simulink model "rtdemo1"  (Simulink 7.8)
settings: Solver=FixedStepDiscrete  StartTime=0.0  StopTime=inf  FixedStep=1  RelTol=1e-3
undefined symbols (not defined in the file or in its folder): j, powergui
libraries: simulink x11, powerlib x9, CampusModeling x5, opal_lib x4, powerlib_extras x3, rtio_opalrt_op5142ex1 x3, rtlab x2
Description:
  | Model of a simple control system for use iin training.
settings Model: Creator=Paul Baracos  LastModifiedBy=wbernal  BufferReuse=off
settings DataIOCC: SaveOutput=off  SaveTime=off  SignalLoggingName=sigsOut
settings OptimizationCC: BlockReduction=off  BooleanDataType=off  InlineInvariantSignals=on  OptimizeBlockIOStorage=off  BufferReuse=off  ExpressionFolding=off  LocalBlockOutputs=off  InitFltsAndDblsToZero=on
settings DebuggingCC: SaveWithParameterizedLinksMsg=none  SignalResolutionControl=TryResolveAllWithWarning  SolverPrmCheckMsg=none  MultiTaskDSMMsg=warning  MultiTaskCondExecSysMsg=none  StrictBusMsg=None
settings HardwareCC: TargetUnknown=on
settings RTWCC: IncludeERTFirstTime=on
settings GRTTargetCC: TargetFcnLib=ansi_tfl_tmw.mat

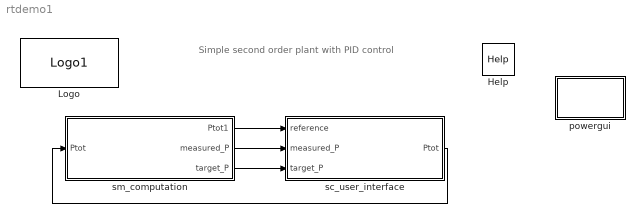
== system rtdemo1 ==
  note: Simple second order plant with PID control
  Help : opal_lib/Help  docfile=../help/help.html
  Logo : opal_lib/Logo1  vide=[]
  powergui : Subsystem  Priority=1  AncestorBlock=powerlib/powergui  InitFcn=powergui( 'InitFcn_Callback' , gcb , 0 , [ ] );  StopFcn=powergui( 'StopFcn_Callback' , gcb , 0 , [ ] );  mask(PSB option menu block){SimulationMode=Phasor, SolverType=Tustin, SampleTime=50e-6, frequency=60, SPID=off, DisableSnubberDevices=off, DisableRonSwitches=off, DisableVfSwitches=off, SwTol=0, Interpol=off, DisplayEquations=off, FunctionMessages=off, frequencyindice=60, Pbase=100e3, ErrMax=1e-4, Iterations=50, UnitsV=kV, UnitsW=MW, echomessages=off, HookPort=off, EnableUseOfTLC=off, x0status=blocks, RestoreLinks=warning, ResistiveCurrentMeasurement=off, Frange=, Ylog=off, Xlog=on, ShowGrid=off, save=off, variable=ZData, structure=, ZoomFFT=off, StartTime=0.0, cycles=1, DisplayStyle=1, fundamental=, FreqAxis=off, MaxFrequency=1000, frequencyindicesteady=1, RmsSteady=, display=off, Ts=, methode=off}
      mask prompts: SimulationMode "Simulation type:"; SolverType "Solver type:"; SampleTime "Sample time (s):"; frequency "Phasor frequency (Hz):"; SPID "Enable use of ideal switching devices"; DisableSnubberDevices "Disable snubbers in switching devices"; DisableRonSwitches "Disable On resistance in switching devices (Ron=0)"; DisableVfSwitches "Disable Forward voltage in switching devices (Vf=0)"; SwTol "Switch tolerance"; Interpol "Interpolate"; DisplayEquations "Display circuit differential equations"; FunctionMessages "Display internal function messages (debug mode feature)"; frequencyindice "Load flow frequency (Hz):"; Pbase "Base power Pbase (VA):"; ErrMax "PQ tolerance (pu):"; Iterations "Max iterations:"; UnitsV "Voltage units"; UnitsW "Power units"; echomessages "Display SimPowerSystems warnings and messages"; HookPort "Add a hook port to the powergui block"; EnableUseOfTLC "Use TLC file when in Accelerator Simulation Mode and for code generation"; x0status "Start simulation with initial electrical states from:"; RestoreLinks "Restore disabled links of SimPowerSystems blocks:"; ResistiveCurrentMeasurement "Use non ideal current measurement blocks (1e-4Ohm internal resistance)"; Frange "Frequency Range"; Ylog "Log impedance"; Xlog "log Frequency"; ShowGrid "grid"; save "Save Data To Workspace"; variable "Variable Name"; structure "Structure Name (PSBFFTSCOPE)"; ZoomFFT "ZoomFFT (PSBFFTSCOPE)"; StartTime "Start Time (PSBFFTSCOPE)"; cycles "Cycles (PSBFFTSCOPE)"; DisplayStyle "Display style (PSBFFTSCOPE)"; fundamental "Fundamental (PSBFFTSCOPE)"; FreqAxis "Frequency Axis (PSBFFTSCOPE)"; MaxFrequency "Max Frequency (PSBFFTSCOPE)"; frequencyindicesteady "Frequency indice (STEADYSTATE)"; RmsSteady "RMS display (STEADYSTATE)"; display "Display Results"; Ts "Old Ts setting (OBSOLETE)"; methode "Phasor simulation (OBSOLETE)"
      mask help: Set simulation type, simulation parameters, and preferences
      mask init:
      | message = powergui('MaskInitialization',gcb,SimulationMode,SampleTime);
      settings: CopyFcn=powergui( 'Copy_Callback' , gcb , 0 , [ ] );  ModelCloseFcn=powergui( 'CloseButton_Callback' , gcb , [ ] , [ ] );  NameChangeFcn=powergui( 'NameChangeFcn_Callback' , gcb , 0 , [ ] );  OpenFcn=powergui(gcb,'Open')
      settings: DeleteFcn=|
      | % see geck 675031 powergui( 'Copy_Callback' , gcb , 1 , [ ] );
      | 
      | powergui( 'CloseButton_Callback' , gcb , [ ] , [ ] );
      settings: PreSaveFcn=|
      | powergui( 'PreSaveFcn_Callback' , gcb , [ ] , [ ] );
      | powergui( 'CloseButton_Callback' , gcb , [ ] , [ ] );
      mask Help: helpview(psbhelp)
      mask StyleString: popup(Continuous|Discrete|Phasor),popup(Tustin|Backward Euler),edit,edit,checkbox,checkbox,checkbox,checkbox,edit,checkbox,checkbox,checkbox,edit,edit,edit,edit,popup(V|kV),popup(W|kW|MW),checkbox,checkbox,checkbox,popup(blocks|steady|zero),popup(yes|warning|no),checkbox,edit,checkbox,checkbox,checkbox,checkbox,edit,edit,checkbox,edit,edit,edit,edit,checkbox,edit,edit,edit,checkbox,edit,checkbox
      mask CallbackString: powergui('SimulationType',[],[],gcb);||||powergui('SPID',[],[],gcb);|||||||||||||||powergui('HookPort',[],[],gcb);|||||||||||||||||||||||
      mask TabNameString: Solver,Solver,Solver,Solver,Solver,Solver,Solver,Solver,Solver,Solver,Solver,Solver,Load Flow,Load Flow,Load Flow,Load Flow,Load Flow,Load Flow,Preferences,Preferences,Preferences,Preferences,Preferences,Preferences,Preferences,Preferences,Preferences,Preferences,Preferences,Preferences,Preferences,Preferences,Preferences,Preferences,Preferences,Preferences,Preferences,Preferences,Preferences,Preferences,Preferences,Solver,Solver
      mask Display: color('blue'),disp(message)
  sc_user_interface : Subsystem
  sm_computation : Subsystem
  wires:
  sc_user_interface/1(Ptot) -> sm_computation/1(Ptot)
  sm_computation/3(target_P) -> sc_user_interface/3(target_P)
  sm_computation/2(measured_P) -> sc_user_interface/2(measured_P)
  sm_computation/1(Ptot1) -> sc_user_interface/1(reference)

== system rtdemo1/powergui ==
  note: Graphical user interface for the analysis of  SimPowerSystems circuits.
      | Place the Powergui block in the top-level of your model and double-click
      | on it to open the GUI.
  EquivalentModel1 : Subsystem
      mask init:
      | SPS = get_param(gcbh,'UserData');
      | if isempty(SPS)
      | 	H=0;
      | 	Rswitch=1;
      | 	InputsNonZero=1;
      | else
      | 	H=SPS.Hswo;
      | 	Rswitch=SPS.Rswitch;
      | 	InputsNonZero=SPS.InputsNonZero;
      | end
      mask Display:
      | color('green')
      | disp('EQUIVALENT CIRCUIT\nPhasor')
  Ground : Ground
  Terminator : Terminator
  wires:
  Ground/1 -> Terminator/1

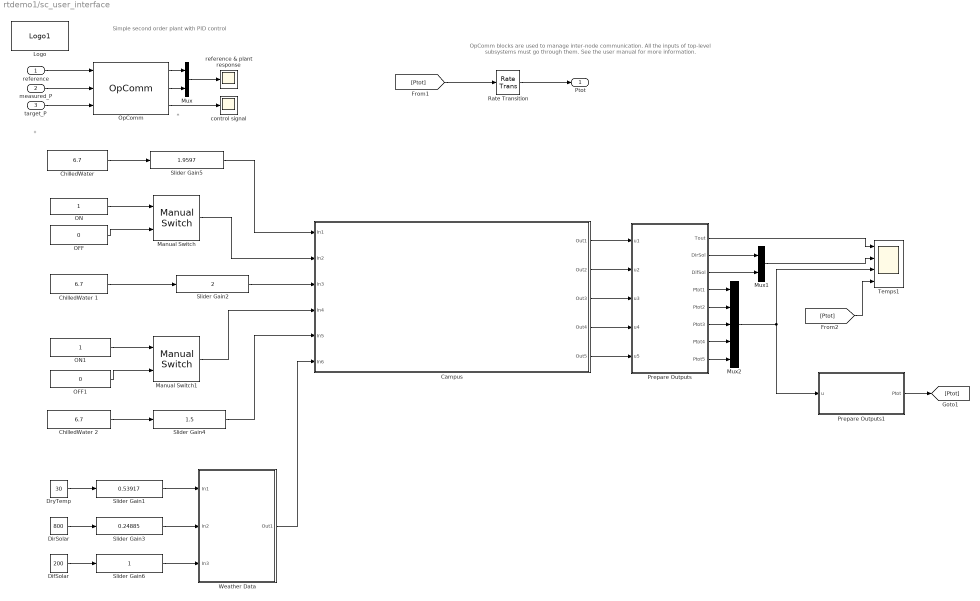
== system rtdemo1/sc_user_interface ==
  note: Simple second order plant with PID control
  note: OpComm blocks are used to manage inter-node communication. All the inputs of top-level
      | subsystems must go through them. See the user manual for more information.
  note: *
  note: *
  reference : Inport
  measured_P : Inport  Port=2
  target_P : Inport  Port=3
  Campus : Subsystem
      mask Display:
      | disp('Campus Model');
      | port_label('input', 1, 'Hospital');
      | port_label('input', 2, 'Secondary School');
      | port_label('input', 3, 'Hospital 1');
      | port_label('input', 4, 'Secondary School');
      | port_label('input', 5, 'Hospital 2');
      | 
      | port_label('output', 1, 'Pout1');
      | % port_label('input', 2, 'int');
      | % port_label('input', 3, 'bool');
      | %a = mfilename('fullpath');
      | %disp(a)
      | image(imread('Campus.jpg'))
  ChilledWater : Constant  Value=6.7
  ChilledWater 1 : Constant  Value=6.7
  ChilledWater 2 : Constant  Value=6.7
  DifSolar : Constant  Value=200
  DirSolar : Constant  Value=800
  DryTemp : Constant  Value=30
  Logo : opal_lib/Logo1  vide=[]
  Manual Switch : simulink/Signal Routing/Manual Switch  sw=0  action=0  varsize=off
  Manual Switch1 : simulink/Signal Routing/Manual Switch  sw=0  action=0  varsize=off
  Mux : Mux  Inputs=2
  Mux1 : Mux  Inputs=2
  Mux2 : Mux  Inputs=5
  OFF : Constant  Value=0
  OFF1 : Constant  Value=0
  ON : Constant
  ON1 : Constant
  OpComm : rtlab/OpComm  nbport=3  groupe_acq=1  subsys_rate=0  st=0  Synchronization=on  Interpolation=on  Threshold=1.0  Missed_Data=off  Sim_Time=off  Samples=off  dynSigOut=off  from_console=0  warning_done=off  writeOpCommFile=off  Offset=off
  Prepare Outputs : MATLAB Function  TreatAsAtomicUnit=on
  Prepare Outputs1 : MATLAB Function  TreatAsAtomicUnit=on
  Rate Transition : RateTransition
  Slider Gain1 : simulink/Math Operations/Slider Gain  low=0.5  gain=0.53917  high=1
  Slider Gain2 : simulink/Math Operations/Slider Gain  low=0.75  gain=2  high=2
  Slider Gain3 : simulink/Math Operations/Slider Gain  low=0  gain=0.24885  high=1
  Slider Gain4 : simulink/Math Operations/Slider Gain  low=0.75  gain=1.5  high=2
  Slider Gain5 : simulink/Math Operations/Slider Gain  low=0.75  gain=1.9597  high=2
  Slider Gain6 : simulink/Math Operations/Slider Gain  low=0  gain=1  high=1
  Temps1 : Scope  NumInputPorts=4
      settings: TimeRange=1883040.935672515  YMin=0~0~0~450000  YMax=21~800~425000~1.45e+006
  Weather Data : Subsystem
  control signal : Scope
      settings: YMin=609462  YMax=673616  SaveName=controlSignal
  reference & plant response : Scope
      settings: Tag=op_tm_save_it  TimeRange=10  YMin=609684  YMax=673862  SaveName=referenceAndPlant
  Ptot : Outport
  wires:
  Mux/1 -> reference & plant response/1
  reference/1 -> OpComm/1
  target_P/1 -> OpComm/3
  measured_P/1 -> OpComm/2
  OpComm/1 -> Mux/1
  OpComm/2 -> Mux/2
  OpComm/3 -> control signal/1
  Campus/1(Out1) -> Prepare Outputs/1(u1)
  Campus/2(Out2) -> Prepare Outputs/2(u2)
  Campus/3(Out3) -> Prepare Outputs/3(u3)
  Campus/4(Out4) -> Prepare Outputs/4(u4)
  Campus/5(Out5) -> Prepare Outputs/5(u5)
  Prepare Outputs/4(Ptot1) -> Mux2/1
  Prepare Outputs/5(Ptot2) -> Mux2/2
  Prepare Outputs/6(Ptot3) -> Mux2/3
  Prepare Outputs/7(Ptot4) -> Mux2/4
  Prepare Outputs/8(Ptot5) -> Mux2/5
  Manual Switch/1 -> Campus/2(In2)
  ChilledWater 1/1 -> Slider Gain2/1
  Slider Gain2/1 -> Campus/3(In3)
  ChilledWater 2/1 -> Slider Gain4/1
  Slider Gain4/1 -> Campus/5(In5)
  ChilledWater/1 -> Slider Gain5/1
  Slider Gain5/1 -> Campus/1(In1)
  ON/1 -> Manual Switch/1
  OFF/1 -> Manual Switch/2
  ON1/1 -> Manual Switch1/1
  OFF1/1 -> Manual Switch1/2
  Manual Switch1/1 -> Campus/4(In4)
  Prepare Outputs1/1(Ptot) -> [Ptot]
  Weather Data/1(Out1) -> Campus/6(In6)
  Prepare Outputs/2(DirSol) -> Mux1/1
  Prepare Outputs/3(DifSol) -> Mux1/2
  Prepare Outputs/1(Tout) -> Temps1/1
  Mux1/1 -> Temps1/2
  Mux2/1 -> Prepare Outputs1/1(u), Temps1/3
  DryTemp/1 -> Slider Gain1/1
  DirSolar/1 -> Slider Gain3/1
  DifSolar/1 -> Slider Gain6/1
  Slider Gain1/1 -> Weather Data/1(In1)
  Slider Gain3/1 -> Weather Data/2(In2)
  Slider Gain6/1 -> Weather Data/3(In3)
  [Ptot] -> Temps1/4
  [Ptot] -> Rate Transition/1
  Rate Transition/1 -> Ptot/1

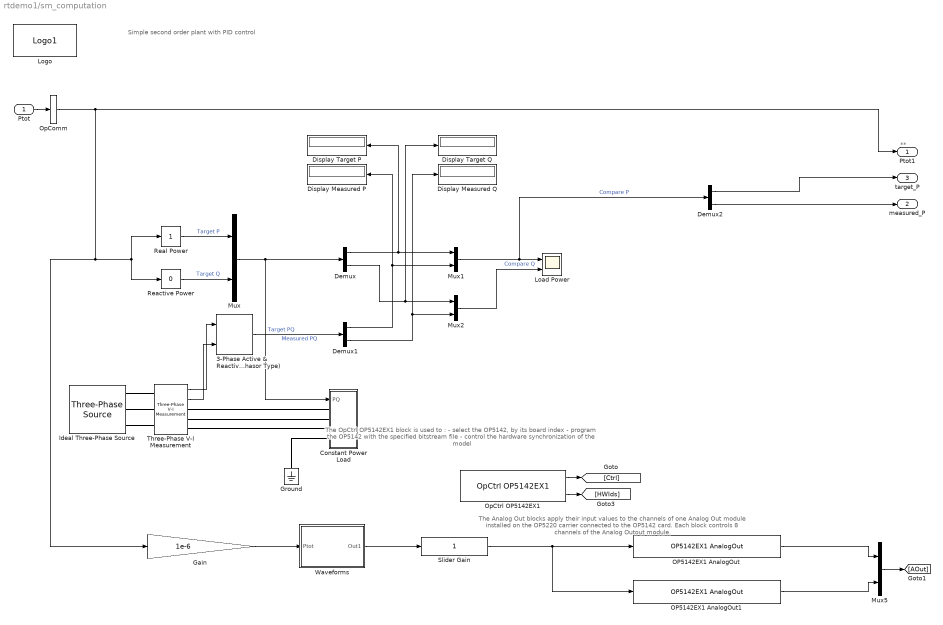
== system rtdemo1/sm_computation ==
  note: Simple second order plant with PID control
  note: **
  note: The OpCtrl OP5142EX1 block is used to :
      | - select the OP5142, by its board index
      | - program the OP5142 with the specified bitstream file
      | - control the hardware synchronization of the model
  note: The Analog Out blocks apply their input values to the channels of one Analog Out module installed on
      | the OP5220 carrier connected to the OP5142 card.
      | Each block controls 8 channels of the Analog Outout module.
  Ptot : Inport
  3-Phase Active & Reactive Power (Phasor Type) : powerlib_extras/Phasor Library/3-Phase Active & Reactive Power (Phasor Type)
  Constant Power Load : Subsystem  mask(Constant Power Load){PNom=5000, QNom=2000, VNom=480, fNom=60, VLow=0.7}
      mask prompts: PNom "Nominal three-phase real power (W)"; QNom "Nominal three-phase reactive power (VAR)"; VNom "Nominal line-to-line voltage (VRMS)"; fNom "Nominal frequency (Hz)"; VLow "Lower voltage limit (pu)"
      mask help: Implements a controllable constant power load, where VI* = P + jQ (in per-unit).
      mask init:
      | % Check voltages
      | if VNom <= 0
      |     error('Nominal line-to-line voltage for a constant power block must be strictly positive.');
      | end
      | if VLow <= 0
      |     error('Lower cutoff voltage for a constant power block must be strictly positive.');
      | end
      mask Help: Implements a controllable constant power load, where VI* = P + jQ (in per-unit).
  Demux : Demux  Outputs=2
  Demux1 : Demux  Outputs=2
  Demux2 : Demux  Outputs=2
  Display Measured P : Display
  Display Measured Q : Display
  Display Target P : Display
  Display Target Q : Display
  Gain : Gain  Gain=1e-6
  Ground : powerlib/Elements/Ground  LConnTagsString=a
  Ideal Three-Phase Source : powerlib/Electrical Sources/Three-Phase Source  Voltage=480  PhaseAngle=0  Frequency=60  InternalConnection=Yg  SpecifyImpedance=on  Resistance=0  Inductance=0  ShortCircuitLevel=100e6  BaseVoltage=480  XRratio=1  BusType=swing  Pref=0  Qref=0  Qmin=-inf  Qmax=inf
  Load Power : Scope  NumInputPorts=2
      settings: TickLabels=on  YMin=2.07616e+006~0  YMax=2.2947e+006~1.5e+006
  Logo : opal_lib/Logo1  vide=[]
  Mux{,1..2,5} (4 alike) : Mux  Inputs=2
  OP5142EX1 AnalogOut : rtio_opalrt_op5142ex1/OP5142EX1 AnalogOut  CtrlName='OP5142EX1 Ctrl'  portNb=1  FcnNos=Slot 1 Module A Subsection 1  size=16  maxcount=8  count=8  numchan=8  israngeinput=off  voltagerange=[-16 ... 16]  slot=0  side=0  mismatch=0  slotside=Slot_1_Module_A
      settings: AttributesFormatString=%<CtrlName>
  OP5142EX1 AnalogOut1 : rtio_opalrt_op5142ex1/OP5142EX1 AnalogOut  CtrlName='OP5142EX1 Ctrl'  portNb=2  FcnNos=Slot 1 Module A Subsection 2  size=16  maxcount=8  count=8  numchan=8  israngeinput=off  voltagerange=[-16 ... 16]  slot=0  side=0  mismatch=0  slotside=Slot_1_Module_A
      settings: AttributesFormatString=%<CtrlName>
  OpComm : rtlab/OpComm  nbport=1  groupe_acq=1  subsys_rate=0  st=0  Synchronization=on  Interpolation=on  Threshold=1.0  Missed_Data=off  Sim_Time=off  Samples=off  dynSigOut=off  from_console=1  warning_done=off  writeOpCommFile=off  Offset=off
  OpCtrl OP5142EX1 : rtio_opalrt_op5142ex1/OpCtrl OP5142EX1  CtrlName='OP5142EX1 Ctrl'  boardid=0  BitstreamFilename=OP5142_1-EX-0000-2_1_3_57-OP5142_8DIO_8TSDIO_6QEIO_16AIO-01-01.bin  numconfig=-1  mode=Master  externalClock=off  decimRtsi=0  calibIO=off  SampleTime=0  loadinport=-1
  Reactive Power : simulink/Math Operations/Slider Gain  low=-5000  gain=0  high=5000
  Real Power : simulink/Math Operations/Slider Gain  low=0  gain=1  high=10000
  Slider Gain : simulink/Math Operations/Slider Gain  low=0  gain=1  high=2
  Three-Phase V-I Measurement : powerlib/Measurements/Three-Phase V-I Measurement  VoltageMeasurement=phase-to-ground  SetLabelV=off  LabelV=Vabc  Vpu=off  VpuLL=off  CurrentMeasurement=yes  SetLabelI=off  LabelI=Iabc  Ipu=off  Pbase=100e6  Vbase=500e3  OutputType=Complex  PhasorSimulation=on  PSBequivalent=0
      link override Model/VI/Ia: GotoTag=LibraryTag_Ia
      link override Model/VI/Ib: GotoTag=LibraryTag_Ib
      link override Model/VI/Ic: GotoTag=LibraryTag_Ic
      link override Model/VI/Va: GotoTag=LibraryTag_Va
      link override Model/VI/Vb: GotoTag=LibraryTag_Vb
      link override Model/VI/Vc: GotoTag=LibraryTag_Vc
  Waveforms : Subsystem
  Ptot1 : Outport
  measured_P : Outport  Port=2
  target_P : Outport  Port=3
  wires:
  Ptot/1 -> OpComm/1
  OpComm/1 -> Ptot1/1, Reactive Power/1, Real Power/1, Gain/1
  Real Power/1 -> Mux/1  "Target P"
  Mux/1 -> Constant Power Load/1(PQ), Demux/1  "Target PQ"
  Three-Phase V-I Measurement/1 -> 3-Phase Active & Reactive Power (Phasor Type)/1
  Three-Phase V-I Measurement/2 -> 3-Phase Active & Reactive Power (Phasor Type)/2
  Reactive Power/1 -> Mux/2  "Target Q"
  3-Phase Active & Reactive Power (Phasor Type)/1 -> Demux1/1  "Measured PQ"
  Mux1/1 -> Load Power/1, Demux2/1  "Compare P"
  Mux2/1 -> Load Power/2  "Compare Q"
  Demux/1 -> Mux1/1, Display Target P/1
  Demux1/1 -> Display Measured P/1, Mux1/2
  Demux/2 -> Mux2/1, Display Target Q/1
  Demux1/2 -> Mux2/2, Display Measured Q/1
  Demux2/1 -> target_P/1
  Demux2/2 -> measured_P/1
  OpCtrl OP5142EX1/1 -> [Ctrl]
  OpCtrl OP5142EX1/2 -> [HWIds]
  OP5142EX1 AnalogOut/1 -> Mux5/1
  OP5142EX1 AnalogOut1/1 -> Mux5/2
  Mux5/1 -> [AOut]
  Slider Gain/1 -> OP5142EX1 AnalogOut/1, OP5142EX1 AnalogOut1/1
  Waveforms/1(Out1) -> Slider Gain/1
  Gain/1 -> Waveforms/1(Ptot)
  connections:
  Constant Power Load/LConn4 -- Ground/LConn1
  Three-Phase V-I Measurement/RConn1 -- Constant Power Load/LConn1
  Three-Phase V-I Measurement/RConn2 -- Constant Power Load/LConn2
  Three-Phase V-I Measurement/RConn3 -- Constant Power Load/LConn3
  Ideal Three-Phase Source/RConn3 -- Three-Phase V-I Measurement/LConn3
  Ideal Three-Phase Source/RConn2 -- Three-Phase V-I Measurement/LConn2
  Ideal Three-Phase Source/RConn1 -- Three-Phase V-I Measurement/LConn1

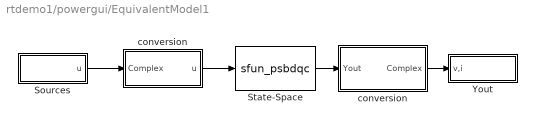
== system rtdemo1/powergui/EquivalentModel1 ==
  Sources : Subsystem
  State-Space : S-Function  FunctionName=sfun_psbdqc  Parameters=real(H), imag(H), Rswitch,InputsNonZero  EnableBusSupport=off
  Yout : Subsystem
  conversion : Subsystem
  "conversion " : Subsystem
  wires:
  State-Space/1 -> conversion/1(Yout)
  conversion/1(Complex) -> Yout/1(v,i)
  "conversion "/1(u) -> State-Space/1
  Sources/1(u) -> "conversion "/1(Complex)

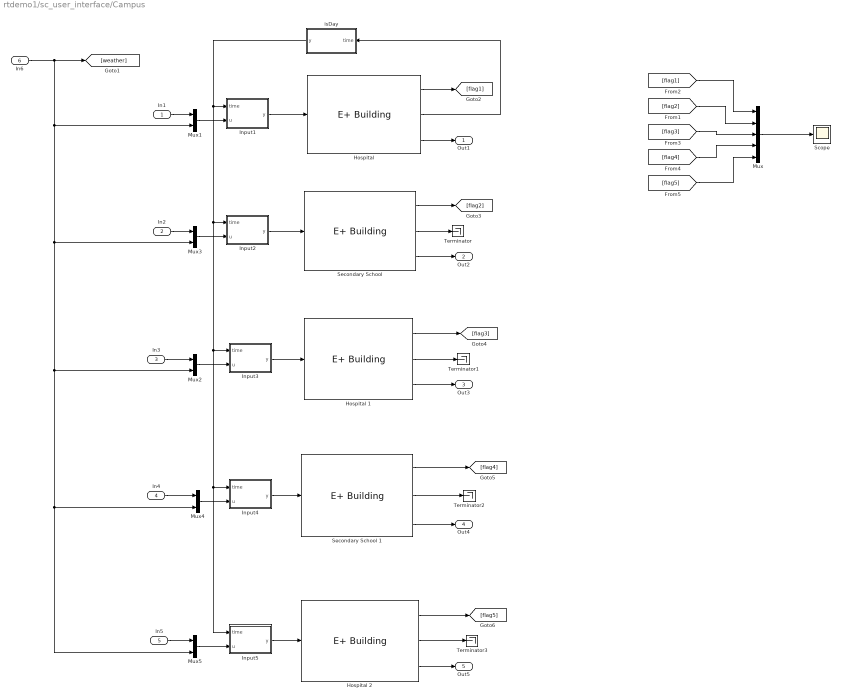
== system rtdemo1/sc_user_interface/Campus ==
  In1 : Inport
  In2 : Inport  Port=2
  In3 : Inport  Port=3
  In4 : Inport  Port=4
  In5 : Inport  Port=5
  In6 : Inport  Port=6
  Hospital : CampusModeling/E+ Building  progname='C:\EnergyPlusV8-0-0-mlep\RunEPlus.bat'  modelfile='U:\CampusModeling\Demo\mlep_campus_rtlab_io\Hospital\RefBldgHospitalNew2004_Chicago'  weatherfile='USA_IL_Chicago-OHare.Intl.AP.725300_TMY3'  workdir='U:\CampusModeling\Demo\mlep_campus_rtlab_io\Hospital'  timeout=200000  port=0  host=''  bcvtbdir=''  deltaT=900  noutputd=12
  Hospital 1 : CampusModeling/E+ Building  progname='C:\EnergyPlusV8-0-0-mlep\RunEPlus.bat'  modelfile='U:\CampusModeling\Demo\mlep_campus_rtlab_io\Hospital1\RefBldgHospitalNew2004_Chicago'  weatherfile='USA_IL_Chicago-OHare.Intl.AP.725300_TMY3'  workdir='U:\CampusModeling\Demo\mlep_campus_rtlab_io\Hospital1'  timeout=200000  port=0  host=''  bcvtbdir=''  deltaT=900  noutputd=12
  Hospital 2 : CampusModeling/E+ Building  progname='C:\EnergyPlusV8-0-0-mlep\RunEPlus.bat'  modelfile='U:\CampusModeling\Demo\mlep_campus_rtlab_io\Hospital2\RefBldgHospitalNew2004_Chicago'  weatherfile='USA_IL_Chicago-OHare.Intl.AP.725300_TMY3'  workdir='U:\CampusModeling\Demo\mlep_campus_rtlab_io\Hospital2'  timeout=200000  port=0  host=''  bcvtbdir=''  deltaT=900  noutputd=12
  Input1 : MATLAB Function  TreatAsAtomicUnit=on
  Input2 : MATLAB Function  TreatAsAtomicUnit=on
  Input3 : MATLAB Function  TreatAsAtomicUnit=on
  Input4 : MATLAB Function  TreatAsAtomicUnit=on
  Input5 : MATLAB Function  TreatAsAtomicUnit=on
  Mux : Mux  Inputs=5
  Mux{1..5} (5 alike) : Mux  Inputs=2
  Scope : Scope
      settings: SaveName=ScopeData2
  Secondary School : CampusModeling/E+ Building  progname='C:\EnergyPlusV8-0-0-mlep\RunEPlus.bat'  modelfile='U:\CampusModeling\Demo\mlep_campus_rtlab_io\SecondarySchool\RefBldgSecondarySchoolNew2004_Chicago'  weatherfile='USA_IL_Chicago-OHare.Intl.AP.725300_TMY3'  workdir='U:\CampusModeling\Demo\mlep_campus_rtlab_io\SecondarySchool'  timeout=200000  port=0  host=''  bcvtbdir=''  deltaT=900  noutputd=21
  Secondary School 1 : CampusModeling/E+ Building  progname='C:\EnergyPlusV8-0-0-mlep\RunEPlus.bat'  modelfile='U:\CampusModeling\Demo\mlep_campus_rtlab_io\SecondarySchool1\RefBldgSecondarySchoolNew2004_Chicago'  weatherfile='USA_IL_Chicago-OHare.Intl.AP.725300_TMY3'  workdir='U:\CampusModeling\Demo\mlep_campus_rtlab_io\SecondarySchool1'  timeout=200000  port=0  host=''  bcvtbdir=''  deltaT=900  noutputd=21
  Terminator{,1..3} (4 alike) : Terminator
  isDay : Subsystem
  Out1 : Outport
  Out2 : Outport  Port=2
  Out3 : Outport  Port=3
  Out4 : Outport  Port=4
  Out5 : Outport  Port=5
  wires:
  Hospital/2 -> isDay/1(time)
  Input1/1(y) -> Hospital/1
  Input2/1(y) -> Secondary School/1
  isDay/1(y) -> Input1/1(time), Input2/1(time), Input3/1(time), Input4/1(time), Input5/1(time)
  Secondary School/2 -> Terminator/1
  Hospital/1 -> [flag1]
  Secondary School/1 -> [flag2]
  Hospital 1/1 -> [flag3]
  Secondary School 1/1 -> [flag4]
  Hospital 2/1 -> [flag5]
  Hospital 1/2 -> Terminator1/1
  Secondary School 1/2 -> Terminator2/1
  Hospital 2/2 -> Terminator3/1
  Input4/1(y) -> Secondary School 1/1
  Input3/1(y) -> Hospital 1/1
  Input5/1(y) -> Hospital 2/1
  Hospital/3 -> Out1/1
  Secondary School/3 -> Out2/1
  Hospital 1/3 -> Out3/1
  Secondary School 1/3 -> Out4/1
  Hospital 2/3 -> Out5/1
  [flag1] -> Mux/1
  [flag2] -> Mux/2
  [flag3] -> Mux/3
  [flag4] -> Mux/4
  [flag5] -> Mux/5
  Mux/1 -> Scope/1
  In6/1 -> [weather], Mux5/2, Mux4/2, Mux2/2, Mux3/2, Mux1/2
  In1/1 -> Mux1/1
  Mux1/1 -> Input1/2(u)
  Mux2/1 -> Input3/2(u)
  In3/1 -> Mux2/1
  In2/1 -> Mux3/1
  Mux3/1 -> Input2/2(u)
  Mux4/1 -> Input4/2(u)
  In4/1 -> Mux4/1
  Mux5/1 -> Input5/2(u)
  In5/1 -> Mux5/1

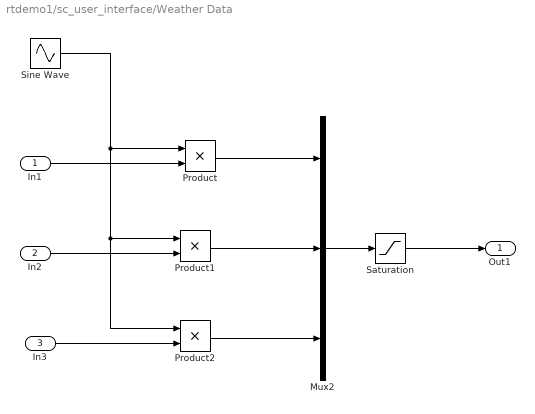
== system rtdemo1/sc_user_interface/Weather Data ==
  In1 : Inport
  In2 : Inport  Port=2
  In3 : Inport  Port=3
  Mux2 : Mux  Inputs=3
  Product : Product  RndMeth=Zero
  Product1 : Product  RndMeth=Zero
  Product2 : Product  RndMeth=Zero
  Saturation : Saturate  UpperLimit=Inf  LowerLimit=0
  Sine Wave : Sin  Frequency=2*pi/(24*60*60)
  Out1 : Outport
  wires:
  Mux2/1 -> Saturation/1
  In1/1 -> Product/2
  Product/1 -> Mux2/1
  Product1/1 -> Mux2/2
  Product2/1 -> Mux2/3
  In2/1 -> Product1/2
  In3/1 -> Product2/2
  Sine Wave/1 -> Product2/1, Product1/1, Product/1
  Saturation/1 -> Out1/1

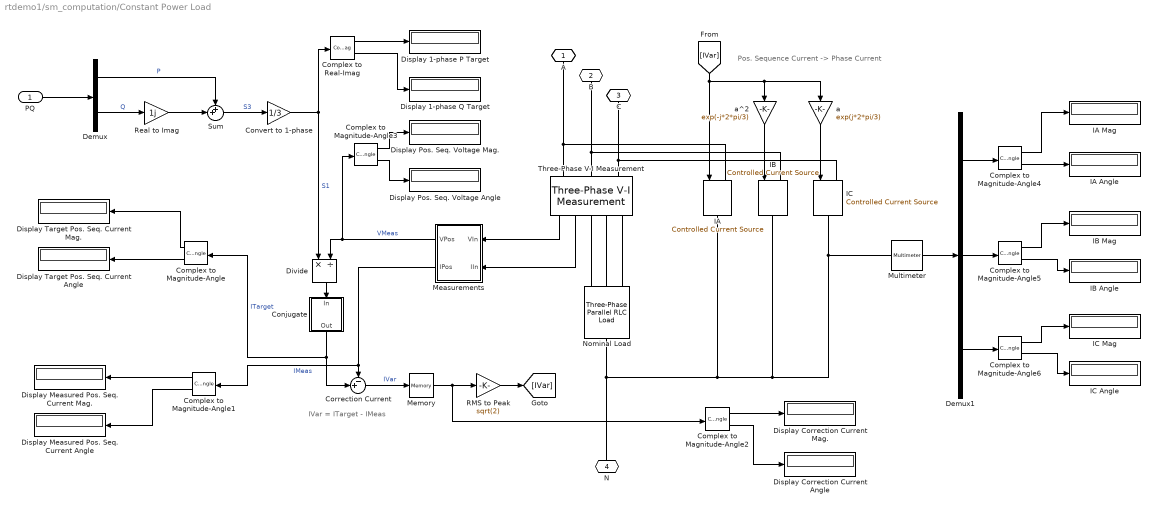
== system rtdemo1/sm_computation/Constant Power Load ==
  note: IVar = ITarget - IMeas
  note: Pos. Sequence Current -> Phase Current
  PQ : Inport  PortDimensions=2
  Complex to Magnitude-Angle{,1..6} (7 alike) : ComplexToMagnitudeAngle
  Complex to Real-Imag : ComplexToRealImag
  Conjugate : Subsystem
  Convert to 1-phase : Gain  Gain=1/3
  Correction Current : Sum  Inputs=-+|
  Demux : Demux  Outputs=2
  Demux1 : Demux  Outputs=3
  Display 1-phase P Target : Display
  Display 1-phase Q Target : Display
  Display Correction Current Angle : Display
  Display Correction Current Mag. : Display
  Display Measured Pos. Seq. Current Angle : Display
  Display Measured Pos. Seq. Current Mag. : Display
  Display Pos. Seq. Voltage Angle : Display
  Display Pos. Seq. Voltage Mag. : Display
  Display Target Pos. Seq. Current Angle : Display
  Display Target Pos. Seq. Current Mag. : Display
  Divide : Product  Inputs=*/
  IA : powerlib/Electrical Sources/Controlled Current Source  Initialize=off  Source_Type=AC  Amplitude=0  Phase=0  Frequency=0  Measurements=Current
  IA Angle : Display
  IA Mag : Display
  IB : powerlib/Electrical Sources/Controlled Current Source  Initialize=off  Source_Type=AC  Amplitude=0  Phase=0  Frequency=0  Measurements=Current
  IB Angle : Display
  IB Mag : Display
  IC : powerlib/Electrical Sources/Controlled Current Source  Initialize=off  Source_Type=AC  Amplitude=0  Phase=0  Frequency=0  Measurements=Current
  IC Angle : Display
  IC Mag : Display
  Measurements : Subsystem
  Memory : Memory
  Multimeter : powerlib/Measurements/Multimeter  PhasorSimulation=on  OutputType=Complex  sel=[1 2 3]  L=3  Gain=[1 1 1]  yselected={'Isrc: sm_computation/Constant Power Load/IA','Isrc: sm_computation/Constant Power Load/IB','Isrc: sm_computation/Constant Power Load/IC'};  PSBOutputType=1  PSBequivalent=0  AxesSetting=[0,0.1,-100,100]  Display=0  SavedBlockNames=-11
  Nominal Load : powerlib/Elements/Three-Phase Parallel RLC Load  LConnTagsString=A|B|C  RConnTagsString=N  Configuration=Y (neutral)  NominalVoltage=VNom  NominalFrequency=fNom  ActivePower=PNom  InductivePower=max(QNom,0)  CapacitivePower=max(-QNom,0)  Measurements=None  LoadType=constant PQ
  RMS to Peak : Gain  Gain=sqrt(2)
  Real to Imag : Gain  Gain=1j
  Sum : Sum  Inputs=++|
  Three-Phase V-I Measurement : powerlib/Measurements/Three-Phase V-I Measurement  VoltageMeasurement=phase-to-ground  SetLabelV=off  LabelV=Vabc  Vpu=off  VpuLL=off  CurrentMeasurement=yes  SetLabelI=off  LabelI=Iabc  Ipu=off  Pbase=100e6  Vbase=VNom  OutputType=Complex  PhasorSimulation=on  PSBequivalent=0
      link override Model/VI/Ia: GotoTag=LibraryTag_Ia
      link override Model/VI/Ib: GotoTag=LibraryTag_Ib
      link override Model/VI/Ic: GotoTag=LibraryTag_Ic
      link override Model/VI/Va: GotoTag=LibraryTag_Va
      link override Model/VI/Vb: GotoTag=LibraryTag_Vb
      link override Model/VI/Vc: GotoTag=LibraryTag_Vc
  a : Gain  Gain=exp(j*2*pi/3)
  a^2 : Gain  Gain=exp(-j*2*pi/3)
  A : PMIOPort  Port=1  Side=Left
  B : PMIOPort  Port=2  Side=Left
  C : PMIOPort  Port=3  Side=Left
  N : PMIOPort  Port=4  Side=Left
  wires:
  Three-Phase V-I Measurement/1 -> Measurements/1(VIn)
  Three-Phase V-I Measurement/2 -> Measurements/2(IIn)
  PQ/1 -> Demux/1
  Demux/2 -> Real to Imag/1  "Q"
  Demux/1 -> Sum/1  "P"
  Real to Imag/1 -> Sum/2
  Measurements/1(VPos) -> Divide/2, Complex to Magnitude-Angle3/1  "VMeas"
  Sum/1 -> Convert to 1-phase/1  "S3"
  Convert to 1-phase/1 -> Divide/1, Complex to Real-Imag/1  "S1"
  Divide/1 -> Conjugate/1(In)
  Measurements/2(IPos) -> Correction Current/1, Complex to Magnitude-Angle1/1  "IMeas"
  [IVar] -> IA/1, a^2/1, a/1
  a^2/1 -> IB/1
  a/1 -> IC/1
  Correction Current/1 -> Memory/1  "IVar"
  Complex to Magnitude-Angle/1 -> Display Target Pos. Seq. Current Mag./1
  Complex to Magnitude-Angle/2 -> Display Target Pos. Seq. Current Angle/1
  Complex to Magnitude-Angle1/1 -> Display Measured Pos. Seq. Current Mag./1
  Complex to Magnitude-Angle1/2 -> Display Measured Pos. Seq. Current Angle/1
  Complex to Magnitude-Angle2/1 -> Display Correction Current Mag./1
  Complex to Magnitude-Angle2/2 -> Display Correction Current Angle/1
  Conjugate/1(Out) -> Correction Current/2, Complex to Magnitude-Angle/1  "ITarget"
  Complex to Real-Imag/1 -> Display 1-phase P Target/1
  Complex to Real-Imag/2 -> Display 1-phase Q Target/1
  Complex to Magnitude-Angle3/1 -> Display Pos. Seq. Voltage Mag./1
  Complex to Magnitude-Angle3/2 -> Display Pos. Seq. Voltage Angle/1
  Demux1/1 -> Complex to Magnitude-Angle4/1
  Complex to Magnitude-Angle4/1 -> IA Mag/1
  Complex to Magnitude-Angle4/2 -> IA Angle/1
  Demux1/2 -> Complex to Magnitude-Angle5/1
  Complex to Magnitude-Angle5/1 -> IB Mag/1
  Complex to Magnitude-Angle5/2 -> IB Angle/1
  Demux1/3 -> Complex to Magnitude-Angle6/1
  Complex to Magnitude-Angle6/1 -> IC Mag/1
  Complex to Magnitude-Angle6/2 -> IC Angle/1
  Multimeter/1 -> Demux1/1
  RMS to Peak/1 -> [IVar]
  Memory/1 -> Complex to Magnitude-Angle2/1, RMS to Peak/1
  connections:
  A/RConn1 -- Three-Phase V-I Measurement/LConn1 -- IA/LConn1
  B/RConn1 -- Three-Phase V-I Measurement/LConn2 -- IB/LConn1
  C/RConn1 -- Three-Phase V-I Measurement/LConn3 -- IC/LConn1
  Three-Phase V-I Measurement/RConn1 -- Nominal Load/LConn1
  Three-Phase V-I Measurement/RConn2 -- Nominal Load/LConn2
  Three-Phase V-I Measurement/RConn3 -- Nominal Load/LConn3
  IB/RConn1 -- IA/RConn1 -- Nominal Load/RConn1 -- N/RConn1 -- IC/RConn1 -- Multimeter/LConn1

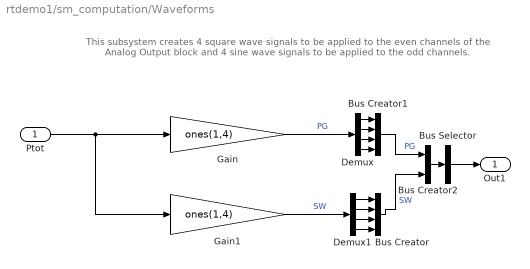
== system rtdemo1/sm_computation/Waveforms ==
  note: This subsystem creates 4 square wave signals to be applied to
      | the even channels of the Analog Output block and 4 sine wave
      | signals to be applied to the odd channels.
  Ptot : Inport
  Bus Creator : BusCreator
  Bus Creator1 : BusCreator
  Bus Creator2 : BusCreator  Inputs=2
  Bus Selector : BusSelector  OutputSignals=PG.signal1,SW.signal1,PG.signal2,SW.signal2,PG.signal3,SW.signal3,PG.signal4,SW.signal4  OutputAsBus=on
  Demux : Demux
  Demux1 : Demux
  Gain : Gain  Gain=ones(1,4)  SaturateOnIntegerOverflow=on  OutDataTypeStr=Inherit: Same as input  ParamDataTypeStr=Inherit: Same as input
  Gain1 : Gain  Gain=ones(1,4)  SaturateOnIntegerOverflow=on  OutDataTypeStr=Inherit: Same as input  ParamDataTypeStr=Inherit: Same as input
  Out1 : Outport
  wires:
  Ptot/1 -> Gain/1, Gain1/1
  Gain/1 -> Demux/1  "PG"
  Bus Creator2/1 -> Bus Selector/1
  Bus Creator1/1 -> Bus Creator2/1  "PG"
  Bus Creator/1 -> Bus Creator2/2  "SW"
  Bus Selector/1 -> Out1/1
  Demux/1 -> Bus Creator1/1
  Demux/2 -> Bus Creator1/2
  Demux/3 -> Bus Creator1/3
  Demux/4 -> Bus Creator1/4
  Gain1/1 -> Demux1/1  "SW"
  Demux1/1 -> Bus Creator/1
  Demux1/2 -> Bus Creator/2
  Demux1/3 -> Bus Creator/3
  Demux1/4 -> Bus Creator/4

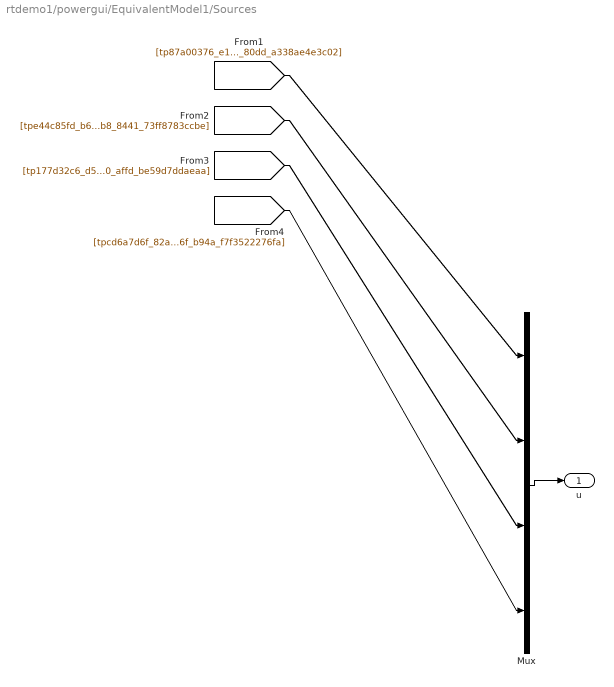
== system rtdemo1/powergui/EquivalentModel1/Sources ==
  Mux : Mux  Inputs=[1 1 1 3]
  u : Outport
  wires:
  Mux/1 -> u/1
  [tp87a00376_e13f_4313_80dd_a338ae4e3c02] -> Mux/1
  [tpe44c85fd_b6e8_42b8_8441_73ff8783ccbe] -> Mux/2
  [tp177d32c6_d55c_4f10_affd_be59d7ddaeaa] -> Mux/3
  [tpcd6a7d6f_82a7_4d6f_b94a_f7f3522276fa] -> Mux/4

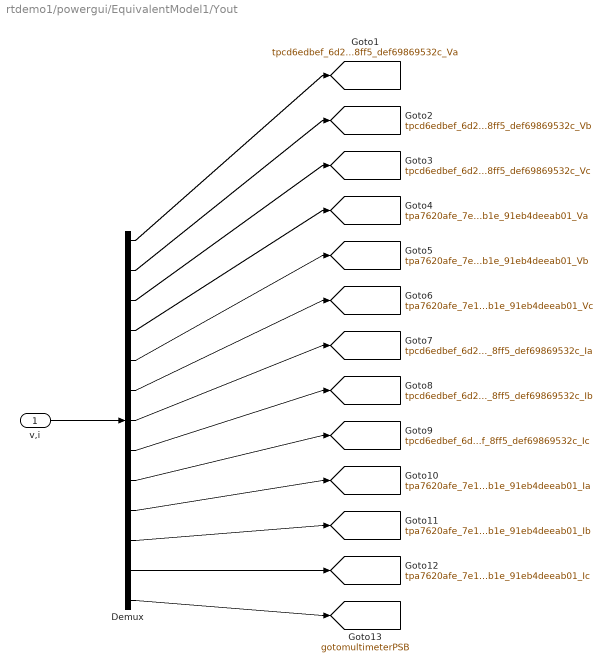
== system rtdemo1/powergui/EquivalentModel1/Yout ==
  v,i : Inport
  Demux : Demux  Outputs=[1 1 1 1 1 1 1 1 1 1 1 1 3]
  tag scope: gotomultimeterPSB=global, tpa7620afe_7e10_40d1_8b1e_91eb4deeab01_Ia=global, tpa7620afe_7e10_40d1_8b1e_91eb4deeab01_Ib=global, tpa7620afe_7e10_40d1_8b1e_91eb4deeab01_Ic=global, tpa7620afe_7e10_40d1_8b1e_91eb4deeab01_Va=global, tpa7620afe_7e10_40d1_8b1e_91eb4deeab01_Vb=global, tpa7620afe_7e10_40d1_8b1e_91eb4deeab01_Vc=global, tpcd6edbef_6d24_43ef_8ff5_def69869532c_Ia=global, tpcd6edbef_6d24_43ef_8ff5_def69869532c_Ib=global, tpcd6edbef_6d24_43ef_8ff5_def69869532c_Ic=global, tpcd6edbef_6d24_43ef_8ff5_def69869532c_Va=global, tpcd6edbef_6d24_43ef_8ff5_def69869532c_Vb=global, tpcd6edbef_6d24_43ef_8ff5_def69869532c_Vc=global
  wires:
  v,i/1 -> Demux/1
  Demux/1 -> [tpcd6edbef_6d24_43ef_8ff5_def69869532c_Va]
  Demux/2 -> [tpcd6edbef_6d24_43ef_8ff5_def69869532c_Vb]
  Demux/3 -> [tpcd6edbef_6d24_43ef_8ff5_def69869532c_Vc]
  Demux/4 -> [tpa7620afe_7e10_40d1_8b1e_91eb4deeab01_Va]
  Demux/5 -> [tpa7620afe_7e10_40d1_8b1e_91eb4deeab01_Vb]
  Demux/6 -> [tpa7620afe_7e10_40d1_8b1e_91eb4deeab01_Vc]
  Demux/7 -> [tpcd6edbef_6d24_43ef_8ff5_def69869532c_Ia]
  Demux/8 -> [tpcd6edbef_6d24_43ef_8ff5_def69869532c_Ib]
  Demux/9 -> [tpcd6edbef_6d24_43ef_8ff5_def69869532c_Ic]
  Demux/10 -> [tpa7620afe_7e10_40d1_8b1e_91eb4deeab01_Ia]
  Demux/11 -> [tpa7620afe_7e10_40d1_8b1e_91eb4deeab01_Ib]
  Demux/12 -> [tpa7620afe_7e10_40d1_8b1e_91eb4deeab01_Ic]
  Demux/13 -> [gotomultimeterPSB]

== system rtdemo1/powergui/EquivalentModel1/conversion ==
  Yout : Inport
  Demux1 : Demux  Outputs=2
  Real-Imag to Complex : RealImagToComplex
  Complex : Outport
  wires:
  Demux1/1 -> Real-Imag to Complex/1
  Demux1/2 -> Real-Imag to Complex/2
  Real-Imag to Complex/1 -> Complex/1
  Yout/1 -> Demux1/1

== system rtdemo1/powergui/EquivalentModel1/conversion  ==
  Complex : Inport
  Complex to Real-Imag : ComplexToRealImag
  Mux : Mux  Inputs=2
  u : Outport
  wires:
  Complex to Real-Imag/1 -> Mux/1
  Complex to Real-Imag/2 -> Mux/2
  Complex/1 -> Complex to Real-Imag/1
  Mux/1 -> u/1

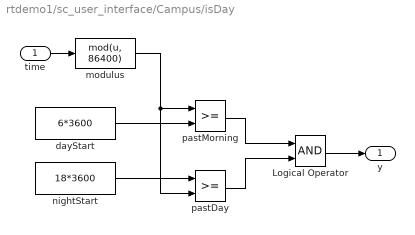
== system rtdemo1/sc_user_interface/Campus/isDay ==
  time : Inport
  Logical Operator : Logic  AllPortsSameDT=off  OutDataTypeStr=boolean
  dayStart : Constant  Value=6*3600
  modulus : MATLABFcn  MATLABFcn=mod(u, 86400)
  nightStart : Constant  Value=18*3600
  pastDay : RelationalOperator  OutDataTypeStr=boolean
  pastMorning : RelationalOperator  OutDataTypeStr=boolean
  y : Outport
  wires:
  time/1 -> modulus/1
  modulus/1 -> pastMorning/1, pastDay/2
  dayStart/1 -> pastMorning/2
  nightStart/1 -> pastDay/1
  pastMorning/1 -> Logical Operator/1
  pastDay/1 -> Logical Operator/2
  Logical Operator/1 -> y/1

== system rtdemo1/sm_computation/Constant Power Load/Conjugate ==
  In : Inport
  Complex to Real-Imag : ComplexToRealImag
  Gain : Gain  Gain=-1
  Real-Imag to Complex : RealImagToComplex
  Out : Outport
  wires:
  In/1 -> Complex to Real-Imag/1
  Complex to Real-Imag/1 -> Real-Imag to Complex/1
  Complex to Real-Imag/2 -> Gain/1
  Gain/1 -> Real-Imag to Complex/2
  Real-Imag to Complex/1 -> Out/1

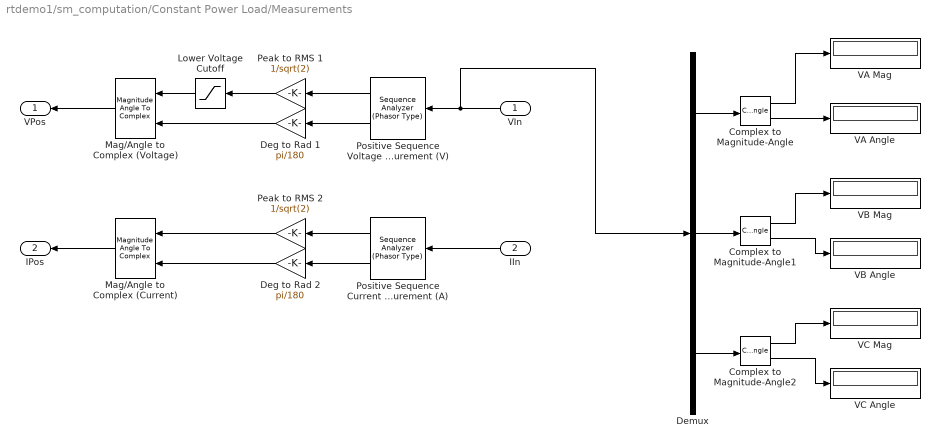
== system rtdemo1/sm_computation/Constant Power Load/Measurements ==
  VIn : Inport
  IIn : Inport  Port=2
  Complex to Magnitude-Angle : ComplexToMagnitudeAngle
  Complex to Magnitude-Angle1 : ComplexToMagnitudeAngle
  Complex to Magnitude-Angle2 : ComplexToMagnitudeAngle
  Deg to Rad 1 : Gain  Gain=pi/180
  Deg to Rad 2 : Gain  Gain=pi/180
  Demux : Demux  Outputs=3
  Lower Voltage Cutoff : Saturate  UpperLimit=inf  LowerLimit=VLow*VNom/sqrt(3)
  Mag/Angle to Complex (Current) : MagnitudeAngleToComplex
  Mag/Angle to Complex (Voltage) : MagnitudeAngleToComplex
  Peak to RMS 1 : Gain  Gain=1/sqrt(2)
  Peak to RMS 2 : Gain  Gain=1/sqrt(2)
  Positive Sequence Current Measurement (A) : powerlib_extras/Phasor Library/Sequence Analyzer (Phasor Type)  seq=Positive
  Positive Sequence Voltage Measurement (V) : powerlib_extras/Phasor Library/Sequence Analyzer (Phasor Type)  seq=Positive
  VA Angle : Display
  VA Mag : Display
  VB Angle : Display
  VB Mag : Display
  VC Angle : Display
  VC Mag : Display
  VPos : Outport
  IPos : Outport  Port=2
  wires:
  Positive Sequence Voltage Measurement (V)/1 -> Peak to RMS 1/1
  Positive Sequence Current Measurement (A)/1 -> Peak to RMS 2/1
  Positive Sequence Current Measurement (A)/2 -> Deg to Rad 2/1
  Lower Voltage Cutoff/1 -> Mag/Angle to Complex (Voltage)/1
  VIn/1 -> Positive Sequence Voltage Measurement (V)/1, Demux/1
  IIn/1 -> Positive Sequence Current Measurement (A)/1
  Mag/Angle to Complex (Voltage)/1 -> VPos/1
  Mag/Angle to Complex (Current)/1 -> IPos/1
  Peak to RMS 1/1 -> Lower Voltage Cutoff/1
  Peak to RMS 2/1 -> Mag/Angle to Complex (Current)/1
  Demux/1 -> Complex to Magnitude-Angle/1
  Complex to Magnitude-Angle/1 -> VA Mag/1
  Complex to Magnitude-Angle/2 -> VA Angle/1
  Demux/2 -> Complex to Magnitude-Angle1/1
  Complex to Magnitude-Angle1/1 -> VB Mag/1
  Complex to Magnitude-Angle1/2 -> VB Angle/1
  Demux/3 -> Complex to Magnitude-Angle2/1
  Complex to Magnitude-Angle2/1 -> VC Mag/1
  Complex to Magnitude-Angle2/2 -> VC Angle/1
  Deg to Rad 1/1 -> Mag/Angle to Complex (Voltage)/2
  Positive Sequence Voltage Measurement (V)/2 -> Deg to Rad 1/1
  Deg to Rad 2/1 -> Mag/Angle to Complex (Current)/2

== matlab function sc_user_interface/Campus/Input2 ==
  data: time input double; u input double; y output double
function y = fcn(time, u)

%% BEGIN - CONTROL
K1 = 0.001;
K2 = 0.0001;

% dayTime = mod(time, 86400);
% if (dayTime >= 6*3600) && (dayTime <= 18*3600)
%     if outputs1(2) + outputs2(2) > 9000
%         change = K1*(outputs1(2) + outputs2(2)-9000);
%         chilledWaterTempSch2 = chilledWaterTempSch2 + change;
%     else
%         change = K2*(outputs1(2) + outputs2(2)-9000);
%         chilledWaterTempSch2 = chilledWaterTempSch2 + change;
%     end
%     if chilledWaterTempSch2 < 7
%         chilledWaterTempSch2 = 7;
%     elseif chilledWaterTempSch2 > 10
%         chilledWaterTempSch2 = 10;
%     end
% end
% 
% 
% 
% inputs1 = [airTempSch roomTempSch chilledWaterTempSch1];
 
y = u;

== matlab function sc_user_interface/Campus/Input1 ==
  data: time input double; u input double; y output double
function y = fcn(time, u)


%% BEGIN - CONTROL
K1 = 0.001;
K2 = 0.0001;

% dayTime = mod(time, 86400);
% if (dayTime >= 6*3600) && (dayTime <= 18*3600)
%     if outputs1(2) + outputs2(2) > 9000
%         change = K1*(outputs1(2) + outputs2(2)-9000);
%         chilledWaterTempSch2 = chilledWaterTempSch2 + change;
%     else
%         change = K2*(outputs1(2) + outputs2(2)-9000);
%         chilledWaterTempSch2 = chilledWaterTempSch2 + change;
%     end
%     if chilledWaterTempSch2 < 7
%         chilledWaterTempSch2 = 7;
%     elseif chilledWaterTempSch2 > 10
%         chilledWaterTempSch2 = 10;
%     end
% end
% 
% 
% 
% inputs1 = [airTempSch roomTempSch chilledWaterTempSch1];
 
y = u;

== matlab function sc_user_interface/Prepare Outputs1 ==
  data: Ptot output double; u input double
function Ptot   = SumPower(u)

Ptot = sum(u(1:end));

== matlab function sc_user_interface/Prepare Outputs ==
  data: Tout output double; DirSol output double; DifSol output double; u1 input double; Ptot1 output double; u2 input double; Ptot2 output double; u3 input double; u4 input double; u5 input double; Ptot3 output double; Ptot4 output double; Ptot5 output double
function [Tout, DirSol, DifSol, Ptot1, Ptot2, Ptot3, Ptot4, Ptot5]  = PrepOutputs(u1, u2, u3, u4, u5)

Tout = u1(1);
DirSol = u1(2);
DifSol = u1(3);

Ptot1 = sum(u1(4:end));
Ptot2 = sum(u2(2:end));
Ptot3 = sum(u3(2:end));
Ptot4 = sum(u4(2:end));
Ptot5 = sum(u5(2:end));

== matlab function sc_user_interface/Campus/Input4 ==
  data: time input double; u input double; y output double
function y = fcn(time, u)


%% BEGIN - CONTROL
K1 = 0.001;
K2 = 0.0001;

% dayTime = mod(time, 86400);
% if (dayTime >= 6*3600) && (dayTime <= 18*3600)
%     if outputs1(2) + outputs2(2) > 9000
%         change = K1*(outputs1(2) + outputs2(2)-9000);
%         chilledWaterTempSch2 = chilledWaterTempSch2 + change;
%     else
%         change = K2*(outputs1(2) + outputs2(2)-9000);
%         chilledWaterTempSch2 = chilledWaterTempSch2 + change;
%     end
%     if chilledWaterTempSch2 < 7
%         chilledWaterTempSch2 = 7;
%     elseif chilledWaterTempSch2 > 10
%         chilledWaterTempSch2 = 10;
%     end
% end
% 
% 
% 
% inputs1 = [airTempSch roomTempSch chilledWaterTempSch1];
 
y = u;

== matlab function sc_user_interface/Campus/Input3 ==
  data: time input double; u input double; y output double
function y = fcn(time, u)


%% BEGIN - CONTROL
K1 = 0.001;
K2 = 0.0001;

% dayTime = mod(time, 86400);
% if (dayTime >= 6*3600) && (dayTime <= 18*3600)
%     if outputs1(2) + outputs2(2) > 9000
%         change = K1*(outputs1(2) + outputs2(2)-9000);
%         chilledWaterTempSch2 = chilledWaterTempSch2 + change;
%     else
%         change = K2*(outputs1(2) + outputs2(2)-9000);
%         chilledWaterTempSch2 = chilledWaterTempSch2 + change;
%     end
%     if chilledWaterTempSch2 < 7
%         chilledWaterTempSch2 = 7;
%     elseif chilledWaterTempSch2 > 10
%         chilledWaterTempSch2 = 10;
%     end
% end
% 
% 
% 
% inputs1 = [airTempSch roomTempSch chilledWaterTempSch1];
 
y = u;

== matlab function sc_user_interface/Campus/Input5 ==
  data: time input double; u input double; y output double
function y = fcn(time, u)


%% BEGIN - CONTROL
K1 = 0.001;
K2 = 0.0001;

% dayTime = mod(time, 86400);
% if (dayTime >= 6*3600) && (dayTime <= 18*3600)
%     if outputs1(2) + outputs2(2) > 9000
%         change = K1*(outputs1(2) + outputs2(2)-9000);
%         chilledWaterTempSch2 = chilledWaterTempSch2 + change;
%     else
%         change = K2*(outputs1(2) + outputs2(2)-9000);
%         chilledWaterTempSch2 = chilledWaterTempSch2 + change;
%     end
%     if chilledWaterTempSch2 < 7
%         chilledWaterTempSch2 = 7;
%     elseif chilledWaterTempSch2 > 10
%         chilledWaterTempSch2 = 10;
%     end
% end
% 
% 
% 
% inputs1 = [airTempSch roomTempSch chilledWaterTempSch1];
 
y = u;
